simulink model "controlGPI_pos_3dof_conMI"  (R2023b)
settings: Solver=VariableStepAuto  StartTime=0.0  StopTime=tsim  FixedStep=1e-5  MaxStep=tstep  RelTol=1e-3
undefined symbols (not defined in the file): contr_robot_params, ddq, dq, MI_Contr1, MI_Contr2, MI_Contr3, MI_motor1, MI_motor2, MI_motor3, ndof, NN_Bspline_params, NN_RBF_params, nn_select, ns, Pc, q, q0, q_cero, q_eq, robot_params, sigbuilder_block, t_qeq_init, t_tr_init, t_trtr, tau_L, tau_L_mags, tr_muestra, Wc, Zc
libraries: mcbcontrolslib x6, spsRMSLib x6, simulink x2
(part 1 of 3)
settings Model: Creator=HP  LastModifiedBy=HP

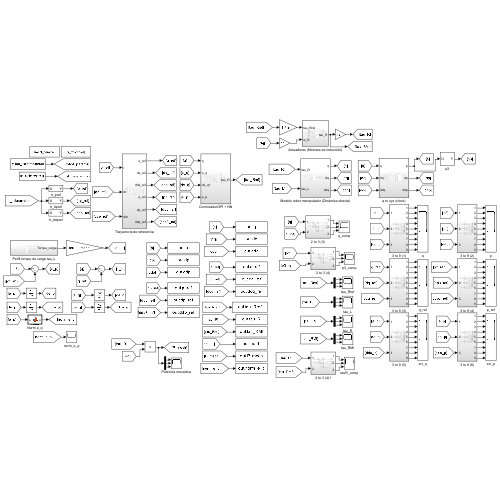
[thumbnail: Simulink's stored preview of the top-level diagram]
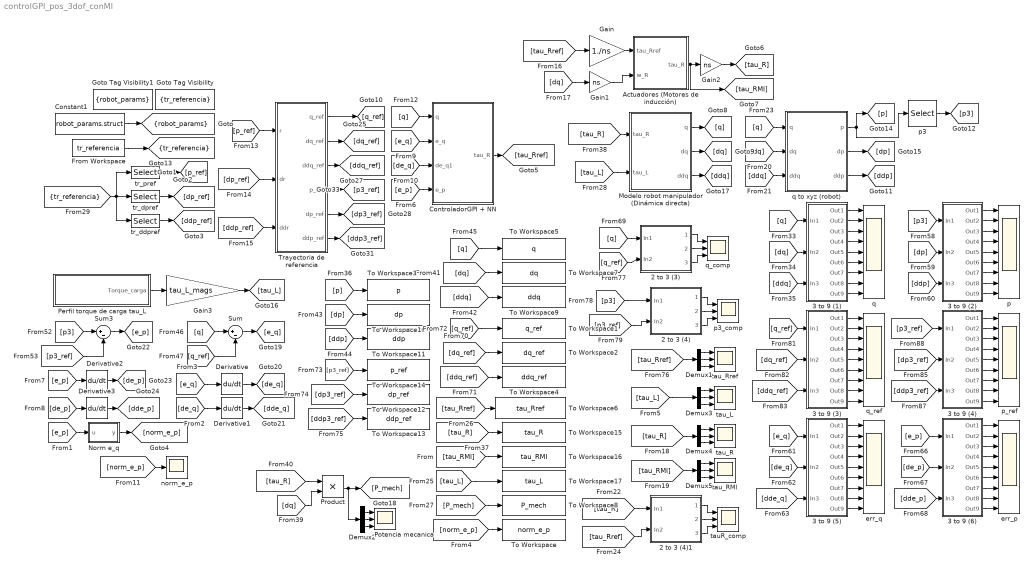
== system controlGPI_pos_3dof_conMI ==
  2 to 3 (3) : Subsystem
  2 to 3 (4) : Subsystem
  2 to 3 (4)1 : Subsystem
  3 to 9 (1) : Subsystem
  3 to 9 (2) : Subsystem
  3 to 9 (3) : Subsystem
  3 to 9 (4) : Subsystem
  3 to 9 (5) : Subsystem
  3 to 9 (6) : Subsystem
  Actuadores (Motores de inducción) : Subsystem
  Constant1 : Constant  Value=robot_params.struct  OutDataTypeStr=Bus: robot_params_bus
  ControladorGPI + NN : Subsystem
  Demux{1..5} (5 alike) : Demux  Outputs=3
  Derivative{,1..3} (4 alike) : Derivative
  From Workspace : FromWorkspace  VariableName=tr_referencia
  Gain : Gain  Gain=1./ns
  Gain1 : Gain  Gain=ns
  Gain2 : Gain  Gain=ns
  Gain3 : Gain  Gain=tau_L_mags
  Goto Tag Visibility : GotoTagVisibility  GotoTag=tr_referencia
  Goto Tag Visibility1 : GotoTagVisibility  GotoTag=robot_params
  Modelo robot manipulador (Dinámica directa) : Subsystem
  Norm e_q : MATLAB Function  TreatAsAtomicUnit=on
  Perfil torque de carga tau_L : Subsystem
  Potencia mecanica : Scope  NumInputPorts=3
  Product : Product
  Sum : Sum  Inputs=|+-
  Sum3 : Sum  Inputs=|+-
  To Workspace : ToWorkspace  VariableName=norm_e_p  SaveFormat=Timeseries  SampleTime=-1
  To Workspace1 : ToWorkspace  VariableName=q_ref  SaveFormat=Timeseries  SampleTime=-1
  To Workspace10 : ToWorkspace  VariableName=dp  SaveFormat=Timeseries  SampleTime=-1
  To Workspace11 : ToWorkspace  VariableName=ddp  SaveFormat=Timeseries  SampleTime=-1
  To Workspace12 : ToWorkspace  VariableName=dp_ref  SaveFormat=Timeseries  SampleTime=-1
  To Workspace13 : ToWorkspace  VariableName=ddp_ref  SaveFormat=Timeseries  SampleTime=-1
  To Workspace14 : ToWorkspace  VariableName=p_ref  SaveFormat=Timeseries  SampleTime=-1
  To Workspace15 : ToWorkspace  VariableName=tau_R  SaveFormat=Timeseries  SampleTime=-1
  To Workspace16 : ToWorkspace  VariableName=tau_RMI  SaveFormat=Timeseries  SampleTime=-1
  To Workspace17 : ToWorkspace  VariableName=tau_L  SaveFormat=Timeseries  SampleTime=-1
  To Workspace2 : ToWorkspace  VariableName=dq_ref  SaveFormat=Timeseries  SampleTime=-1
  To Workspace3 : ToWorkspace  VariableName=p  SaveFormat=Timeseries  SampleTime=-1
  To Workspace4 : ToWorkspace  VariableName=ddq_ref  SaveFormat=Timeseries  SampleTime=-1
  To Workspace5 : ToWorkspace  VariableName=q  SaveFormat=Timeseries  SampleTime=-1
  To Workspace6 : ToWorkspace  VariableName=tau_Rref  SaveFormat=Timeseries  SampleTime=-1
  To Workspace7 : ToWorkspace  VariableName=dq  SaveFormat=Timeseries  SampleTime=-1
  To Workspace8 : ToWorkspace  VariableName=P_mech  SaveFormat=Timeseries  SampleTime=-1
  To Workspace9 : ToWorkspace  VariableName=ddq  SaveFormat=Timeseries  SampleTime=-1
  Trayectoria de referencia : Subsystem
  err_p : Scope  NumInputPorts=9
  err_q : Scope  NumInputPorts=9
  norm_e_p : Scope
  p : Scope  NumInputPorts=9
  p3 : Selector  NumberOfDimensions=2  InputPortWidth=3  IndexOptions=Index vector (dialog),Index vector (dialog)  Indices=[1:3],3  OutputSizes=1,1
  p3_comp : Scope  NumInputPorts=3
  p_ref : Scope  NumInputPorts=9
  q : Scope  NumInputPorts=9
  q to xyz (robot) : Subsystem
  q_comp : Scope  NumInputPorts=3
  q_ref : Scope  NumInputPorts=9
  tauR_comp : Scope  NumInputPorts=3
  tau_L : Scope  NumInputPorts=3
  tau_R : Scope  NumInputPorts=3
  tau_RMI : Scope  NumInputPorts=3
  tau_Rref : Scope  NumInputPorts=3
  tr_ddpref : Selector  NumberOfDimensions=2  InputPortWidth=3  IndexOptions=Index vector (dialog),Index vector (dialog)  Indices=[7:9],1  OutputSizes=1,1
  tr_dpref : Selector  NumberOfDimensions=2  InputPortWidth=3  IndexOptions=Index vector (dialog),Index vector (dialog)  Indices=[4:6],1  OutputSizes=1,1
  tr_pref : Selector  NumberOfDimensions=2  InputPortWidth=3  IndexOptions=Index vector (dialog),Index vector (dialog)  Indices=[1:3],1  OutputSizes=1,1
  tag scope: robot_params=scoped, tr_referencia=scoped
  wires:
  From Workspace/1 -> [tr_referencia]
  Constant1/1 -> [robot_params]
  [tau_L] -> Modelo robot manipulador (Dinámica directa)/2(tau_L)
  [tau_R] -> Modelo robot manipulador (Dinámica directa)/1(tau_R)
  Modelo robot manipulador (Dinámica directa)/1(q) -> [q]
  Modelo robot manipulador (Dinámica directa)/2(dq) -> [dq]
  Modelo robot manipulador (Dinámica directa)/3(ddq) -> [ddq]
  [tr_referencia] -> tr_ddpref/1, tr_pref/1, tr_dpref/1
  tr_pref/1 -> [p_ref]
  tr_dpref/1 -> [dp_ref]
  tr_ddpref/1 -> [ddp_ref]
  3 to 9 (6)/4(Out4) -> err_p/4
  [e_q] -> 3 to 9 (5)/1(In1)
  3 to 9 (5)/6(Out6) -> err_q/6
  3 to 9 (5)/3(Out3) -> err_q/3
  3 to 9 (3)/6(Out6) -> q_ref/6
  3 to 9 (4)/4(Out4) -> p_ref/4
  Demux1/3 -> tau_Rref/3
  3 to 9 (5)/8(Out8) -> err_q/8
  [dq_ref] -> 3 to 9 (3)/2(In2)
  [dq] -> 3 to 9 (1)/2(In2)
  2 to 3 (4)/1(1) -> p3_comp/1
  3 to 9 (2)/6(Out6) -> p/6
  [tau_R] -> Product/1
  Product/1 -> Demux2/1, [P_mech]
  [q] -> 3 to 9 (1)/1(In1)
  3 to 9 (2)/3(Out3) -> p/3
  3 to 9 (1)/9(Out9) -> q/9
  [p3] -> 2 to 3 (4)/1(In1)
  2 to 3 (3)/2(2) -> q_comp/2
  [ddq_ref] -> 3 to 9 (3)/3(In3)
  3 to 9 (1)/5(Out5) -> q/5
  3 to 9 (3)/7(Out7) -> q_ref/7
  3 to 9 (2)/1(Out1) -> p/1
  3 to 9 (6)/1(Out1) -> err_p/1
  Demux2/1 -> Potencia mecanica/1
  3 to 9 (5)/9(Out9) -> err_q/9
  3 to 9 (3)/5(Out5) -> q_ref/5
  [dde_p] -> 3 to 9 (6)/3(In3)
  3 to 9 (5)/2(Out2) -> err_q/2
  3 to 9 (6)/8(Out8) -> err_p/8
  [p3] -> 3 to 9 (2)/1(In1)
  2 to 3 (3)/3(3) -> q_comp/3
  [tau_L] -> Demux3/1
  Demux2/2 -> Potencia mecanica/2
  3 to 9 (2)/2(Out2) -> p/2
  Demux1/2 -> tau_Rref/2
  3 to 9 (1)/6(Out6) -> q/6
  [de_q] -> 3 to 9 (5)/2(In2)
  3 to 9 (4)/6(Out6) -> p_ref/6
  [e_p] -> 3 to 9 (6)/1(In1)
  2 to 3 (4)/2(2) -> p3_comp/2
  3 to 9 (4)/7(Out7) -> p_ref/7
  3 to 9 (6)/5(Out5) -> err_p/5
  3 to 9 (4)/2(Out2) -> p_ref/2
  [dq] -> Product/2
  3 to 9 (1)/1(Out1) -> q/1
  3 to 9 (3)/8(Out8) -> q_ref/8
  3 to 9 (2)/9(Out9) -> p/9
  3 to 9 (3)/1(Out1) -> q_ref/1
  [de_p] -> 3 to 9 (6)/2(In2)
  [q] -> 2 to 3 (3)/1(In1)
  3 to 9 (1)/7(Out7) -> q/7
  3 to 9 (1)/2(Out2) -> q/2
  [q_ref] -> 2 to 3 (3)/2(In2)
  [tau_Rref] -> Demux1/1
  [ddq] -> 3 to 9 (1)/3(In3)
  3 to 9 (6)/2(Out2) -> err_p/2
  3 to 9 (4)/9(Out9) -> p_ref/9
  3 to 9 (5)/1(Out1) -> err_q/1
  3 to 9 (2)/4(Out4) -> p/4
  3 to 9 (2)/7(Out7) -> p/7
  3 to 9 (3)/4(Out4) -> q_ref/4
  3 to 9 (5)/7(Out7) -> err_q/7
  3 to 9 (4)/1(Out1) -> p_ref/1
  [p3_ref] -> 2 to 3 (4)/2(In2)
  [dde_q] -> 3 to 9 (5)/3(In3)
  3 to 9 (4)/8(Out8) -> p_ref/8
  3 to 9 (6)/6(Out6) -> err_p/6
  3 to 9 (1)/4(Out4) -> q/4
  3 to 9 (3)/3(Out3) -> q_ref/3
  3 to 9 (3)/9(Out9) -> q_ref/9
  2 to 3 (3)/1(1) -> q_comp/1
  3 to 9 (4)/5(Out5) -> p_ref/5
  [q_ref] -> 3 to 9 (3)/1(In1)
  2 to 3 (4)/3(3) -> p3_comp/3
  [dp3_ref] -> 3 to 9 (4)/2(In2)
  3 to 9 (1)/8(Out8) -> q/8
  [ddp3_ref] -> 3 to 9 (4)/3(In3)
  3 to 9 (5)/4(Out4) -> err_q/4
  3 to 9 (3)/2(Out2) -> q_ref/2
  3 to 9 (2)/5(Out5) -> p/5
  3 to 9 (5)/5(Out5) -> err_q/5
  3 to 9 (4)/3(Out3) -> p_ref/3
  Demux2/3 -> Potencia mecanica/3
  [p3_ref] -> 3 to 9 (4)/1(In1)
  3 to 9 (6)/3(Out3) -> err_p/3
  3 to 9 (2)/8(Out8) -> p/8
  3 to 9 (6)/9(Out9) -> err_p/9
  [ddp] -> 3 to 9 (2)/3(In3)
  [dp] -> 3 to 9 (2)/2(In2)
  Demux1/1 -> tau_Rref/1
  3 to 9 (1)/3(Out3) -> q/3
  3 to 9 (6)/7(Out7) -> err_p/7
  q to xyz (robot)/1(p) -> p3/1, [p]
  [dq] -> q to xyz (robot)/2(dq)
  [ddq] -> q to xyz (robot)/3(ddq)
  [q] -> To Workspace5/1
  [dq_ref] -> To Workspace2/1
  [q] -> q to xyz (robot)/1(q)
  [ddq] -> To Workspace9/1
  [p3_ref] -> To Workspace14/1
  [ddq_ref] -> To Workspace4/1
  [q_ref] -> To Workspace1/1
  q to xyz (robot)/2(dp) -> [dp]
  [dp] -> To Workspace10/1
  [dp3_ref] -> To Workspace12/1
  q to xyz (robot)/3(ddp) -> [ddp]
  [ddp] -> To Workspace11/1
  [p] -> To Workspace3/1
  [dq] -> To Workspace7/1
  p3/1 -> [p3]
  [ddp3_ref] -> To Workspace13/1
  [norm_e_p] -> norm_e_p/1
  Derivative2/1 -> [de_p]
  [e_p] -> Derivative2/1
  Derivative3/1 -> [dde_p]
  Derivative1/1 -> [dde_q]
  [e_q] -> Derivative/1
  [de_p] -> Derivative3/1
  Norm e_q/1(y) -> [norm_e_p]
  [e_p] -> Norm e_q/1(u)
  [p3_ref] -> Sum3/2
  Sum/1 -> [e_q]
  [de_q] -> Derivative1/1
  [q_ref] -> Sum/2
  [q] -> Sum/1
  Derivative/1 -> [de_q]
  [p3] -> Sum3/1
  Sum3/1 -> [e_p]
  [e_q] -> ControladorGPI + NN/2(e_q)
  [e_p] -> ControladorGPI + NN/4(e_p)
  [q] -> ControladorGPI + NN/1(q)
  [de_q] -> ControladorGPI + NN/3(de_q1)
  ControladorGPI + NN/1(tau_R) -> [tau_Rref]
  Demux3/3 -> tau_L/3
  Demux3/2 -> tau_L/2
  Demux3/1 -> tau_L/1
  [p_ref] -> Trayectoria de referencia/1(r)
  Trayectoria de referencia/6(ddp_ref) -> [ddp3_ref]
  Trayectoria de referencia/2(dq_ref) -> [dq_ref]
  [dp_ref] -> Trayectoria de referencia/2(dr)
  Trayectoria de referencia/5(dp_ref) -> [dp3_ref]
  Trayectoria de referencia/1(q_ref) -> [q_ref]
  Trayectoria de referencia/4(p_ref) -> [p3_ref]
  Trayectoria de referencia/3(ddq_ref) -> [ddq_ref]
  [ddp_ref] -> Trayectoria de referencia/3(ddr)
  Gain/1 -> Actuadores (Motores de inducción)/1(tau_Rref)
  Actuadores (Motores de inducción)/1(tau_R) -> [tau_RMI], Gain2/1
  Gain1/1 -> Actuadores (Motores de inducción)/2(w_R)
  Gain2/1 -> [tau_R]
  [tau_Rref] -> Gain/1
  [dq] -> Gain1/1
  Demux4/3 -> tau_R/3
  Demux4/1 -> tau_R/1
  Demux4/2 -> tau_R/2
  [tau_R] -> Demux4/1
  [tau_RMI] -> Demux5/1
  Demux5/2 -> tau_RMI/2
  Demux5/3 -> tau_RMI/3
  Demux5/1 -> tau_RMI/1
  2 to 3 (4)1/3(3) -> tauR_comp/3
  2 to 3 (4)1/2(2) -> tauR_comp/2
  2 to 3 (4)1/1(1) -> tauR_comp/1
  [tau_R] -> 2 to 3 (4)1/1(In1)
  [tau_Rref] -> 2 to 3 (4)1/2(In2)
  Perfil torque de carga tau_L/1(Torque_carga) -> Gain3/1
  Gain3/1 -> [tau_L]
  [P_mech] -> To Workspace8/1
  [tau_Rref] -> To Workspace6/1
  [tau_RMI] -> To Workspace16/1
  [tau_R] -> To Workspace15/1
  [tau_L] -> To Workspace17/1
  [norm_e_p] -> To Workspace/1

== system controlGPI_pos_3dof_conMI/2 to 3 (3) ==
  In1 : Inport
  In2 : Inport  Port=2
  Demux3 : Demux  Outputs=3
  Demux4 : Demux  Outputs=3
  Mux10 : Mux  Inputs=2
  Mux8 : Mux  Inputs=2
  Mux9 : Mux  Inputs=2
  1 : Outport
  2 : Outport  Port=2
  3 : Outport  Port=3
  wires:
  Demux4/3 -> Mux10/2
  Demux3/1 -> Mux8/1
  Demux3/2 -> Mux9/1
  Mux9/1 -> 2/1
  Demux4/2 -> Mux9/2
  Demux4/1 -> Mux8/2
  Demux3/3 -> Mux10/1
  Mux8/1 -> 1/1
  Mux10/1 -> 3/1
  In1/1 -> Demux3/1
  In2/1 -> Demux4/1

== system controlGPI_pos_3dof_conMI/2 to 3 (4) ==
  In1 : Inport
  In2 : Inport  Port=2
  Demux3 : Demux  Outputs=3
  Demux4 : Demux  Outputs=3
  Mux10 : Mux  Inputs=2
  Mux8 : Mux  Inputs=2
  Mux9 : Mux  Inputs=2
  1 : Outport
  2 : Outport  Port=2
  3 : Outport  Port=3
  wires:
  Demux4/3 -> Mux10/2
  Demux3/1 -> Mux8/1
  Demux3/2 -> Mux9/1
  Mux9/1 -> 2/1
  Demux4/2 -> Mux9/2
  Demux4/1 -> Mux8/2
  Demux3/3 -> Mux10/1
  Mux8/1 -> 1/1
  Mux10/1 -> 3/1
  In1/1 -> Demux3/1
  In2/1 -> Demux4/1

== system controlGPI_pos_3dof_conMI/2 to 3 (4)1 ==
  In1 : Inport
  In2 : Inport  Port=2
  Demux3 : Demux  Outputs=3
  Demux4 : Demux  Outputs=3
  Mux10 : Mux  Inputs=2
  Mux8 : Mux  Inputs=2
  Mux9 : Mux  Inputs=2
  1 : Outport
  2 : Outport  Port=2
  3 : Outport  Port=3
  wires:
  Demux4/3 -> Mux10/2
  Demux3/1 -> Mux8/1
  Demux3/2 -> Mux9/1
  Mux9/1 -> 2/1
  Demux4/2 -> Mux9/2
  Demux4/1 -> Mux8/2
  Demux3/3 -> Mux10/1
  Mux8/1 -> 1/1
  Mux10/1 -> 3/1
  In1/1 -> Demux3/1
  In2/1 -> Demux4/1

== system controlGPI_pos_3dof_conMI/3 to 9 (1) ==
  In1 : Inport
  In2 : Inport  Port=2
  In3 : Inport  Port=3
  Demux2 : Demux  Outputs=3
  Demux3 : Demux  Outputs=3
  Demux4 : Demux  Outputs=3
  Out1 : Outport
  Out2 : Outport  Port=2
  Out3 : Outport  Port=3
  Out4 : Outport  Port=4
  Out5 : Outport  Port=5
  Out6 : Outport  Port=6
  Out7 : Outport  Port=7
  Out8 : Outport  Port=8
  Out9 : Outport  Port=9
  wires:
  In3/1 -> Demux4/1
  Demux4/1 -> Out3/1
  Demux2/1 -> Out1/1
  Demux3/3 -> Out8/1
  Demux3/2 -> Out5/1
  Demux3/1 -> Out2/1
  In1/1 -> Demux2/1
  Demux2/3 -> Out7/1
  Demux4/3 -> Out9/1
  Demux4/2 -> Out6/1
  Demux2/2 -> Out4/1
  In2/1 -> Demux3/1

== system controlGPI_pos_3dof_conMI/3 to 9 (2) ==
  In1 : Inport
  In2 : Inport  Port=2
  In3 : Inport  Port=3
  Demux2 : Demux  Outputs=3
  Demux3 : Demux  Outputs=3
  Demux4 : Demux  Outputs=3
  Out1 : Outport
  Out2 : Outport  Port=2
  Out3 : Outport  Port=3
  Out4 : Outport  Port=4
  Out5 : Outport  Port=5
  Out6 : Outport  Port=6
  Out7 : Outport  Port=7
  Out8 : Outport  Port=8
  Out9 : Outport  Port=9
  wires:
  In3/1 -> Demux4/1
  Demux4/1 -> Out3/1
  Demux2/1 -> Out1/1
  Demux3/3 -> Out8/1
  Demux3/2 -> Out5/1
  Demux3/1 -> Out2/1
  In1/1 -> Demux2/1
  Demux2/3 -> Out7/1
  Demux4/3 -> Out9/1
  Demux4/2 -> Out6/1
  Demux2/2 -> Out4/1
  In2/1 -> Demux3/1

== system controlGPI_pos_3dof_conMI/3 to 9 (3) ==
  In1 : Inport
  In2 : Inport  Port=2
  In3 : Inport  Port=3
  Demux2 : Demux  Outputs=3
  Demux3 : Demux  Outputs=3
  Demux4 : Demux  Outputs=3
  Out1 : Outport
  Out2 : Outport  Port=2
  Out3 : Outport  Port=3
  Out4 : Outport  Port=4
  Out5 : Outport  Port=5
  Out6 : Outport  Port=6
  Out7 : Outport  Port=7
  Out8 : Outport  Port=8
  Out9 : Outport  Port=9
  wires:
  In3/1 -> Demux4/1
  Demux4/1 -> Out3/1
  Demux2/1 -> Out1/1
  Demux3/3 -> Out8/1
  Demux3/2 -> Out5/1
  Demux3/1 -> Out2/1
  In1/1 -> Demux2/1
  Demux2/3 -> Out7/1
  Demux4/3 -> Out9/1
  Demux4/2 -> Out6/1
  Demux2/2 -> Out4/1
  In2/1 -> Demux3/1

== system controlGPI_pos_3dof_conMI/3 to 9 (4) ==
  In1 : Inport
  In2 : Inport  Port=2
  In3 : Inport  Port=3
  Demux2 : Demux  Outputs=3
  Demux3 : Demux  Outputs=3
  Demux4 : Demux  Outputs=3
  Out1 : Outport
  Out2 : Outport  Port=2
  Out3 : Outport  Port=3
  Out4 : Outport  Port=4
  Out5 : Outport  Port=5
  Out6 : Outport  Port=6
  Out7 : Outport  Port=7
  Out8 : Outport  Port=8
  Out9 : Outport  Port=9
  wires:
  In3/1 -> Demux4/1
  Demux4/1 -> Out3/1
  Demux2/1 -> Out1/1
  Demux3/3 -> Out8/1
  Demux3/2 -> Out5/1
  Demux3/1 -> Out2/1
  In1/1 -> Demux2/1
  Demux2/3 -> Out7/1
  Demux4/3 -> Out9/1
  Demux4/2 -> Out6/1
  Demux2/2 -> Out4/1
  In2/1 -> Demux3/1

== system controlGPI_pos_3dof_conMI/3 to 9 (5) ==
  In1 : Inport
  In2 : Inport  Port=2
  In3 : Inport  Port=3
  Demux2 : Demux  Outputs=3
  Demux3 : Demux  Outputs=3
  Demux4 : Demux  Outputs=3
  Out1 : Outport
  Out2 : Outport  Port=2
  Out3 : Outport  Port=3
  Out4 : Outport  Port=4
  Out5 : Outport  Port=5
  Out6 : Outport  Port=6
  Out7 : Outport  Port=7
  Out8 : Outport  Port=8
  Out9 : Outport  Port=9
  wires:
  In3/1 -> Demux4/1
  Demux4/1 -> Out3/1
  Demux2/1 -> Out1/1
  Demux3/3 -> Out8/1
  Demux3/2 -> Out5/1
  Demux3/1 -> Out2/1
  In1/1 -> Demux2/1
  Demux2/3 -> Out7/1
  Demux4/3 -> Out9/1
  Demux4/2 -> Out6/1
  Demux2/2 -> Out4/1
  In2/1 -> Demux3/1

== system controlGPI_pos_3dof_conMI/3 to 9 (6) ==
  In1 : Inport
  In2 : Inport  Port=2
  In3 : Inport  Port=3
  Demux2 : Demux  Outputs=3
  Demux3 : Demux  Outputs=3
  Demux4 : Demux  Outputs=3
  Out1 : Outport
  Out2 : Outport  Port=2
  Out3 : Outport  Port=3
  Out4 : Outport  Port=4
  Out5 : Outport  Port=5
  Out6 : Outport  Port=6
  Out7 : Outport  Port=7
  Out8 : Outport  Port=8
  Out9 : Outport  Port=9
  wires:
  In3/1 -> Demux4/1
  Demux4/1 -> Out3/1
  Demux2/1 -> Out1/1
  Demux3/3 -> Out8/1
  Demux3/2 -> Out5/1
  Demux3/1 -> Out2/1
  In1/1 -> Demux2/1
  Demux2/3 -> Out7/1
  Demux4/3 -> Out9/1
  Demux4/2 -> Out6/1
  Demux2/2 -> Out4/1
  In2/1 -> Demux3/1

== system controlGPI_pos_3dof_conMI/Actuadores (Motores de inducción) ==
  tau_Rref : Inport
  w_R : Inport  Port=2
  Demux : Demux  Outputs=3
  Demux3 : Demux  Outputs=3
  MI1 + PBC Torque Controller : Subsystem
  MI2 + PBC Torque Controller : Subsystem
  MI3 + PBC Torque Controller : Subsystem
  Mux : Mux  Inputs=3
  tau_R : Outport
  wires:
  Demux3/1 -> MI1 + PBC Torque Controller/2(dq)
  Demux/1 -> MI1 + PBC Torque Controller/1(tau_Rref)
  MI1 + PBC Torque Controller/1(tau_R) -> Mux/1
  Demux3/3 -> MI3 + PBC Torque Controller/2(dq)
  MI2 + PBC Torque Controller/1(tau_R) -> Mux/2
  MI3 + PBC Torque Controller/1(tau_R) -> Mux/3
  Demux3/2 -> MI2 + PBC Torque Controller/2(dq)
  Demux/3 -> MI3 + PBC Torque Controller/1(tau_Rref)
  Demux/2 -> MI2 + PBC Torque Controller/1(tau_Rref)
  tau_Rref/1 -> Demux/1
  w_R/1 -> Demux3/1
  Mux/1 -> tau_R/1

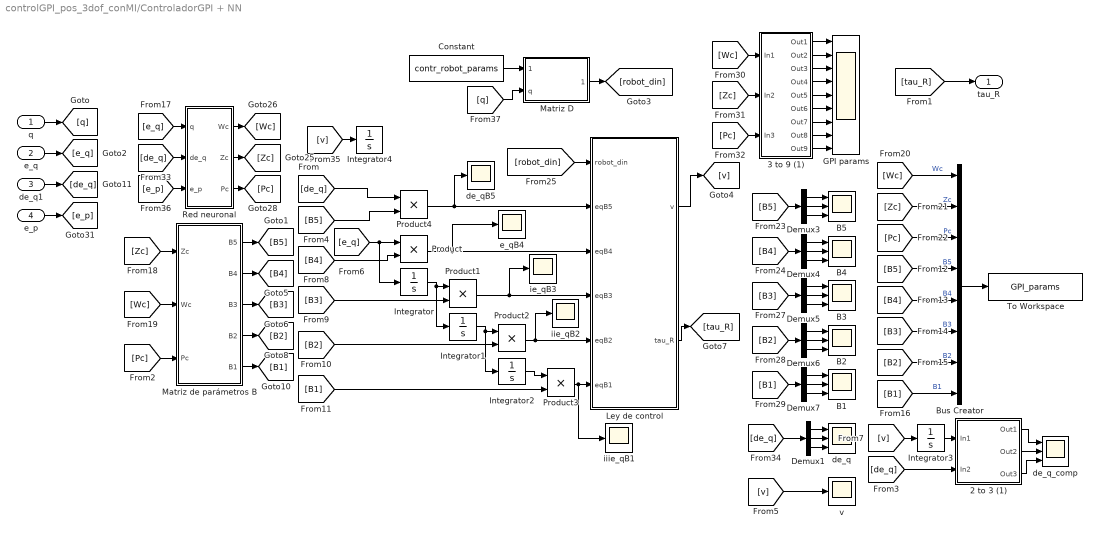
== system controlGPI_pos_3dof_conMI/ControladorGPI + NN ==
  q : Inport
  e_q : Inport  Port=2
  de_q1 : Inport  Port=3
  e_p : Inport  Port=4
  2 to 3 (1) : Subsystem
  3 to 9 (1) : Subsystem
  B{1..5} (5 alike) : Scope  NumInputPorts=3
  Bus Creator : BusCreator  Inputs=8
  Constant : Constant  Value=contr_robot_params  OutDataTypeStr=Bus: robot_params_bus
  Demux{1,3..7} (6 alike) : Demux  Outputs=3
  GPI params : Scope  NumInputPorts=9
  Integrator{,1..4} (5 alike) : Integrator
  Ley de control : MATLAB Function  TreatAsAtomicUnit=on
  Matriz D : MATLAB Function  TreatAsAtomicUnit=on
  Matriz de parámetros B : MATLAB Function  TreatAsAtomicUnit=on
  Product{,1..4} (5 alike) : Product
  Red neuronal : Subsystem
  To Workspace : ToWorkspace  VariableName=GPI_params  SaveFormat=Timeseries  SampleTime=-1
  de_q : Scope  NumInputPorts=3
  de_qB5 : Scope
  de_q_comp : Scope  NumInputPorts=3
  e_qB4 : Scope
  ie_qB3 : Scope
  iie_qB2 : Scope
  iiie_qB1 : Scope
  v : Scope
  tau_R : Outport
  wires:
  Ley de control/2(tau_R) -> [tau_R]
  [tau_R] -> tau_R/1
  e_q/1 -> [e_q]
  [e_q] -> Integrator/1, Product/1
  Integrator/1 -> Integrator1/1, Product1/1
  Integrator1/1 -> Integrator2/1, Product2/1
  Integrator2/1 -> Product3/1
  Product3/1 -> iiie_qB1/1, Ley de control/6(eqB1)
  Product2/1 -> iie_qB2/1, Ley de control/5(eqB2)
  Product1/1 -> ie_qB3/1, Ley de control/4(eqB3)
  Product/1 -> e_qB4/1, Ley de control/3(eqB4)
  Ley de control/1(v) -> [v]
  Product4/1 -> de_qB5/1, Ley de control/2(eqB5)
  [Zc] -> Matriz de parámetros B/1(Zc)
  [Wc] -> Matriz de parámetros B/2(Wc)
  [Pc] -> Matriz de parámetros B/3(Pc)
  Matriz de parámetros B/1(B5) -> [B5]
  Matriz de parámetros B/2(B4) -> [B4]
  Matriz de parámetros B/3(B3) -> [B3]
  Matriz de parámetros B/4(B2) -> [B2]
  Matriz de parámetros B/5(B1) -> [B1]
  [B5] -> Product4/2
  [B4] -> Product/2
  [B3] -> Product1/2
  [B2] -> Product2/2
  [B1] -> Product3/2
  Bus Creator/1 -> To Workspace/1
  [Wc] -> Bus Creator/1  "Wc"
  [Zc] -> Bus Creator/2  "Zc"
  [Pc] -> Bus Creator/3  "Pc"
  [B5] -> Bus Creator/4  "B5"
  [B4] -> Bus Creator/5  "B4"
  [B3] -> Bus Creator/6  "B3"
  [B2] -> Bus Creator/7  "B2"
  [B1] -> Bus Creator/8  "B1"
  Demux3/2 -> B5/2
  Demux3/1 -> B5/1
  [B5] -> Demux3/1
  Demux4/2 -> B4/2
  Demux4/1 -> B4/1
  [B4] -> Demux4/1
  Demux5/1 -> B3/1
  Demux5/2 -> B3/2
  [B3] -> Demux5/1
  Demux6/1 -> B2/1
  Demux6/2 -> B2/2
  [B2] -> Demux6/1
  Demux7/1 -> B1/1
  Demux7/2 -> B1/2
  [B1] -> Demux7/1
  Red neuronal/2(Zc) -> [Zc]
  Red neuronal/1(Wc) -> [Wc]
  Red neuronal/3(Pc) -> [Pc]
  [de_q] -> Red neuronal/2(de_q)
  [e_q] -> Red neuronal/1(q)
  [de_q] -> Demux1/1
  Demux1/1 -> de_q/1
  Demux1/2 -> de_q/2
  de_q1/1 -> [de_q]
  e_p/1 -> [e_p]
  [e_p] -> Red neuronal/3(e_p)
  [robot_din] -> Ley de control/1(robot_din)
  q/1 -> [q]
  [v] -> Integrator3/1
  Integrator3/1 -> 2 to 3 (1)/1(In1)
  [de_q] -> 2 to 3 (1)/2(In2)
  [v] -> v/1
  [v] -> Integrator4/1
  [de_q] -> Product4/1
  3 to 9 (1)/6(Out6) -> GPI params/6
  3 to 9 (1)/9(Out9) -> GPI params/9
  3 to 9 (1)/2(Out2) -> GPI params/2
  3 to 9 (1)/8(Out8) -> GPI params/8
  [Pc] -> 3 to 9 (1)/3(In3)
  3 to 9 (1)/1(Out1) -> GPI params/1
  [Wc] -> 3 to 9 (1)/1(In1)
  3 to 9 (1)/7(Out7) -> GPI params/7
  3 to 9 (1)/4(Out4) -> GPI params/4
  3 to 9 (1)/3(Out3) -> GPI params/3
  [Zc] -> 3 to 9 (1)/2(In2)
  3 to 9 (1)/5(Out5) -> GPI params/5
  2 to 3 (1)/1(Out1) -> de_q_comp/1
  2 to 3 (1)/2(Out2) -> de_q_comp/2
  2 to 3 (1)/3(Out3) -> de_q_comp/3
  Demux3/3 -> B5/3
  Demux4/3 -> B4/3
  Demux5/3 -> B3/3
  Demux6/3 -> B2/3
  Demux7/3 -> B1/3
  Demux1/3 -> de_q/3
  Constant/1 -> Matriz D/1(robot_params)
  [q] -> Matriz D/2(q)
  Matriz D/1(robot_din) -> [robot_din]

== system controlGPI_pos_3dof_conMI/Modelo robot manipulador (Dinámica directa) ==
  tau_R : Inport
  tau_L : Inport  Port=2
  Dinámica directa : MATLAB Function  TreatAsAtomicUnit=on
  int_ddq : Integrator  InitialCondition=q_cero
  int_dq : Integrator  InitialCondition=q_eq
  q : Outport
  dq : Outport  Port=2
  ddq : Outport  Port=3
  wires:
  [tau_L] -> Dinámica directa/5(tau_L)
  int_ddq/1 -> [dq], int_dq/1
  [robot_params] -> Dinámica directa/1(robot_params)
  [dq] -> Dinámica directa/3(dq)
  int_dq/1 -> [q]
  [tau_R] -> Dinámica directa/4(tau_R)
  Dinámica directa/1(ddq) -> int_ddq/1, [ddq]
  [q] -> q/1
  [dq] -> dq/1
  [ddq] -> ddq/1
  tau_R/1 -> [tau_R]
  tau_L/1 -> [tau_L]
  [q] -> Dinámica directa/2(q)

== system controlGPI_pos_3dof_conMI/Perfil torque de carga tau_L ==
  Bus Selector : BusSelector  OutputSignals=sel_perfil
  Bus Selector1 : BusSelector  OutputSignals=sel_perfil
  Constant17 : Constant  Value=tau_L.perfiles  OutDataTypeStr=Bus: Perfil_bus
  If : If  IfExpression=u1 == 1  ElseIfExpressions=u1 == 2,u1 == 3,u1 == 4,u1 == 5,u1 == 6,u1 == 7,u1 == 8
  If Action Subsystem : Subsystem  TreatAsAtomicUnit=on
  If Action Subsystem1 : Subsystem  TreatAsAtomicUnit=on
  If Action Subsystem2 : Subsystem  TreatAsAtomicUnit=on
  If Action Subsystem3 : Subsystem  TreatAsAtomicUnit=on
  If Action Subsystem4 : Subsystem  TreatAsAtomicUnit=on
  If Action Subsystem5 : Subsystem  TreatAsAtomicUnit=on
  If Action Subsystem6 : Subsystem  TreatAsAtomicUnit=on
  If Action Subsystem7 : Subsystem  TreatAsAtomicUnit=on
  tau_L : MultiPortSwitch  Inputs=9  SaturateOnIntegerOverflow=off  InputSameDT=off
  Torque_carga : Outport
  wires:
  tau_L/1 -> Torque_carga/1
  [ramp] -> tau_L/4
  [trEsca] -> tau_L/7
  [pol7] -> tau_L/6
  [sen] -> tau_L/5
  [esca] -> tau_L/3
  Constant17/1 -> [perfil_params]
  [ts] -> tau_L/8
  [tr15segs] -> tau_L/9
  Bus Selector/1 -> tau_L/1  "<sel_perfil>"
  [perfil_params] -> Bus Selector/1
  If Action Subsystem/1(sen) -> [sen]
  [perfil_params] -> Bus Selector1/1
  Bus Selector1/1 -> If/1  "<sel_perfil>"
  If/4 -> If Action Subsystem/Action
  If Action Subsystem1/1(cero) -> [cero]
  [cero] -> tau_L/2
  [perfil_params] -> If Action Subsystem/1(perfil_params)
  If/1 -> If Action Subsystem1/Action
  If Action Subsystem2/1(esca) -> [esca]
  If/2 -> If Action Subsystem2/Action
  If Action Subsystem3/1(ramp) -> [ramp]
  If/3 -> If Action Subsystem3/Action
  [perfil_params] -> If Action Subsystem4/1(perfil_params)
  If/5 -> If Action Subsystem4/Action
  If Action Subsystem4/1(pol7) -> [pol7]
  If Action Subsystem5/1(trEsca) -> [trEsca]
  [perfil_params] -> If Action Subsystem5/1(perfil_params)
  If Action Subsystem6/1(ts) -> [ts]
  If/6 -> If Action Subsystem5/Action
  If/7 -> If Action Subsystem6/Action
  If Action Subsystem7/1(tr15segs) -> [tr15segs]
  If/8 -> If Action Subsystem7/Action
  [perfil_params] -> If Action Subsystem7/1(perfil_params)

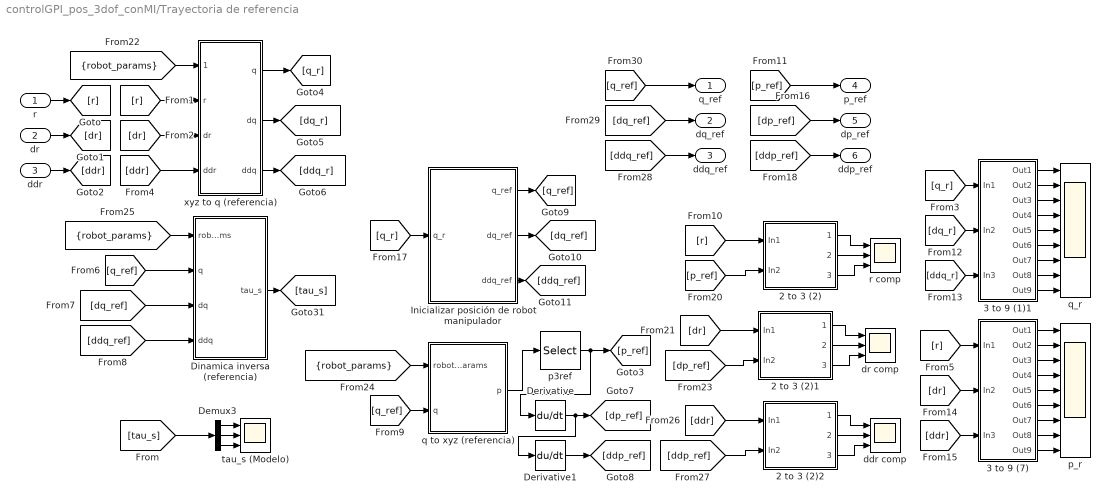
== system controlGPI_pos_3dof_conMI/Trayectoria de referencia ==
  r : Inport
  dr : Inport  Port=2
  ddr : Inport  Port=3
  2 to 3 (2) : Subsystem
  2 to 3 (2)1 : Subsystem
  2 to 3 (2)2 : Subsystem
  3 to 9 (1)1 : Subsystem
  3 to 9 (7) : Subsystem
  Demux3 : Demux  Outputs=3
  Derivative : Derivative
  Derivative1 : Derivative
  Dinamica inversa (referencia) : MATLAB Function  TreatAsAtomicUnit=on
  Inicializar posición de robot manipulador : Subsystem
  ddr comp : Scope  NumInputPorts=3
  dr comp : Scope  NumInputPorts=3
  p3ref : Selector  NumberOfDimensions=2  InputPortWidth=3  IndexOptions=Index vector (dialog),Index vector (dialog)  Indices=[1:3],3  OutputSizes=1,1
  p_r : Scope  NumInputPorts=9
  q to xyz (referencia) : MATLAB Function  TreatAsAtomicUnit=on
  q_r : Scope  NumInputPorts=9
  r comp : Scope  NumInputPorts=3
  tau_s (Modelo) : Scope  NumInputPorts=3
  xyz to q (referencia) : MATLAB Function  TreatAsAtomicUnit=on
  q_ref : Outport
  dq_ref : Outport  Port=2
  ddq_ref : Outport  Port=3
  p_ref : Outport  Port=4
  dp_ref : Outport  Port=5
  ddp_ref : Outport  Port=6
  wires:
  xyz to q (referencia)/1(q) -> [q_r]
  [robot_params] -> xyz to q (referencia)/1(robot_params)
  [dq_ref] -> Dinamica inversa (referencia)/3(dq)
  [q_ref] -> Dinamica inversa (referencia)/2(q)
  [q_ref] -> q to xyz (referencia)/2(q)
  [r] -> xyz to q (referencia)/2(r)
  xyz to q (referencia)/2(dq) -> [dq_r]
  q to xyz (referencia)/1(p) -> p3ref/1
  [robot_params] -> Dinamica inversa (referencia)/1(robot_params)
  Dinamica inversa (referencia)/1(tau_s) -> [tau_s]
  xyz to q (referencia)/3(ddq) -> [ddq_r]
  [ddq_ref] -> Dinamica inversa (referencia)/4(ddq)
  [ddr] -> xyz to q (referencia)/4(ddr)
  [dr] -> xyz to q (referencia)/3(dr)
  r/1 -> [r]
  dr/1 -> [dr]
  ddr/1 -> [ddr]
  Derivative/1 -> Derivative1/1, [dp_ref]
  [tau_s] -> Demux3/1
  [q_r] -> Inicializar posición de robot manipulador/1(q_r)
  [robot_params] -> q to xyz (referencia)/1(robot_params)
  2 to 3 (2)/2(2) -> r comp/2
  p3ref/1 -> [p_ref], Derivative/1
  2 to 3 (2)/1(1) -> r comp/1
  [r] -> 2 to 3 (2)/1(In1)
  2 to 3 (2)/3(3) -> r comp/3
  [p_ref] -> p_ref/1
  Derivative1/1 -> [ddp_ref]
  [dp_ref] -> dp_ref/1
  [ddp_ref] -> ddp_ref/1
  [p_ref] -> 2 to 3 (2)/2(In2)
  [dp_ref] -> 2 to 3 (2)1/2(In2)
  2 to 3 (2)1/2(2) -> dr comp/2
  2 to 3 (2)1/1(1) -> dr comp/1
  [dr] -> 2 to 3 (2)1/1(In1)
  2 to 3 (2)1/3(3) -> dr comp/3
  [ddp_ref] -> 2 to 3 (2)2/2(In2)
  2 to 3 (2)2/2(2) -> ddr comp/2
  2 to 3 (2)2/1(1) -> ddr comp/1
  [ddr] -> 2 to 3 (2)2/1(In1)
  2 to 3 (2)2/3(3) -> ddr comp/3
  Inicializar posición de robot manipulador/1(q_ref) -> [q_ref]
  Inicializar posición de robot manipulador/2(dq_ref) -> [dq_ref]
  Inicializar posición de robot manipulador/3(ddq_ref) -> [ddq_ref]
  [ddq_ref] -> ddq_ref/1
  [dq_ref] -> dq_ref/1
  [q_ref] -> q_ref/1
  3 to 9 (7)/4(Out4) -> p_r/4
  3 to 9 (7)/5(Out5) -> p_r/5
  3 to 9 (7)/8(Out8) -> p_r/8
  [ddr] -> 3 to 9 (7)/3(In3)
  [dq_r] -> 3 to 9 (1)1/2(In2)
  3 to 9 (7)/1(Out1) -> p_r/1
  3 to 9 (1)1/5(Out5) -> q_r/5
  3 to 9 (1)1/3(Out3) -> q_r/3
  3 to 9 (7)/3(Out3) -> p_r/3
  [r] -> 3 to 9 (7)/1(In1)
  3 to 9 (1)1/4(Out4) -> q_r/4
  3 to 9 (1)1/6(Out6) -> q_r/6
  [q_r] -> 3 to 9 (1)1/1(In1)
  3 to 9 (1)1/8(Out8) -> q_r/8
  3 to 9 (7)/7(Out7) -> p_r/7
  3 to 9 (1)1/7(Out7) -> q_r/7
  3 to 9 (1)1/1(Out1) -> q_r/1
  3 to 9 (1)1/2(Out2) -> q_r/2
  [dr] -> 3 to 9 (7)/2(In2)
  3 to 9 (7)/6(Out6) -> p_r/6
  3 to 9 (7)/2(Out2) -> p_r/2
  3 to 9 (7)/9(Out9) -> p_r/9
  3 to 9 (1)1/9(Out9) -> q_r/9
  [ddq_r] -> 3 to 9 (1)1/3(In3)
  Demux3/2 -> tau_s (Modelo)/2
  Demux3/1 -> tau_s (Modelo)/1
  Demux3/3 -> tau_s (Modelo)/3

== system controlGPI_pos_3dof_conMI/q to xyz (robot) ==
  q : Inport
  dq : Inport  Port=2
  ddq : Inport  Port=3
  Data Store Memory : DataStoreMemory  DataStoreName=q  WriteAfterWriteMsg=warning  InitialValue=zeros(size(q(:,1)))  ShowAdditionalParam=off
  Data Store Memory1 : DataStoreMemory  DataStoreName=dq  WriteAfterWriteMsg=warning  InitialValue=zeros(size(dq(:,1)))  ShowAdditionalParam=off
  Data Store Memory2 : DataStoreMemory  DataStoreName=ddq  WriteAfterWriteMsg=warning  InitialValue=zeros(size(ddq(:,1)))  ShowAdditionalParam=off
  Data Store Read : DataStoreRead  DataStoreName=q  IndexOptions=Index vector (dialog)  Indices=1  OutputSizes=1
  Data Store Read1 : DataStoreRead  DataStoreName=dq  IndexOptions=Index vector (dialog)  Indices=1  OutputSizes=1
  Data Store Read2 : DataStoreRead  DataStoreName=ddq  IndexOptions=Index vector (dialog)  Indices=1  OutputSizes=1
  Data Store Write : DataStoreWrite  DataStoreName=q  IndexOptions=Index vector (dialog)  Indices=1  OutputSizes=1
  Data Store Write1 : DataStoreWrite  DataStoreName=dq  IndexOptions=Index vector (dialog)  Indices=1  OutputSizes=1
  Data Store Write2 : DataStoreWrite  DataStoreName=ddq  IndexOptions=Index vector (dialog)  Indices=1  OutputSizes=1
  q to xyz (referencia) : MATLAB Function  TreatAsAtomicUnit=on
  p : Outport
  dp : Outport  Port=2
  ddp : Outport  Port=3
  wires:
  q/1 -> Data Store Write/1
  ddq/1 -> Data Store Write2/1
  dq/1 -> Data Store Write1/1
  Data Store Read/1 -> q to xyz (referencia)/2(q)
  Data Store Read1/1 -> q to xyz (referencia)/3(dq)
  Data Store Read2/1 -> q to xyz (referencia)/4(ddq)
  q to xyz (referencia)/1(p) -> p/1
  q to xyz (referencia)/2(dp) -> dp/1
  q to xyz (referencia)/3(ddp) -> ddp/1
  [robot_params] -> q to xyz (referencia)/1(robot_params)

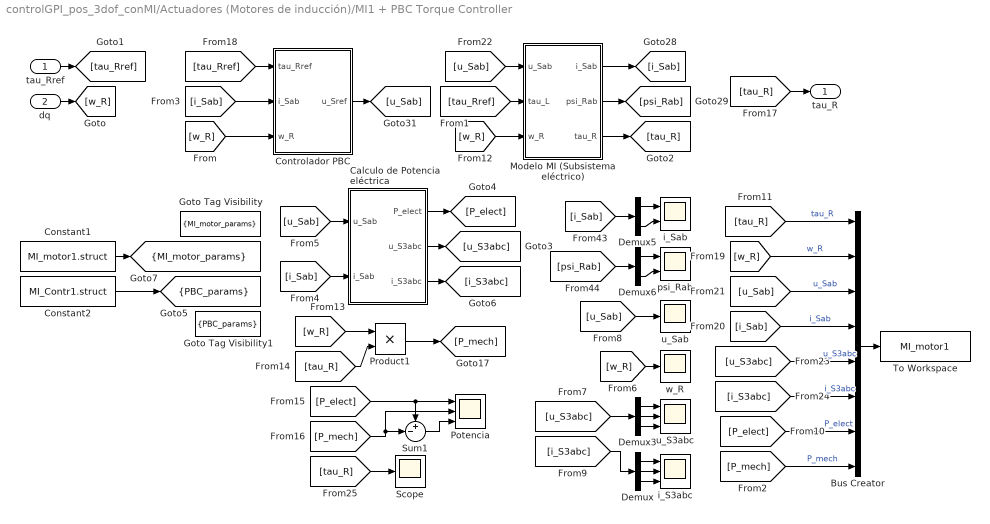
== system controlGPI_pos_3dof_conMI/Actuadores (Motores de inducción)/MI1 + PBC Torque Controller ==
  tau_Rref : Inport
  dq : Inport  Port=2
  Bus Creator : BusCreator  Inputs=8
  Calculo de Potencia eléctrica : Subsystem
  Constant1 : Constant  Value=MI_motor1.struct  OutDataTypeStr=Bus: MI_bus
  Constant2 : Constant  Value=MI_Contr1.struct  OutDataTypeStr=Bus: PBC_bus
  Controlador PBC : Subsystem
  Demux : Demux  Outputs=3
  Demux3 : Demux  Outputs=3
  Demux5 : Demux  Outputs=2
  Demux6 : Demux  Outputs=2
  Goto Tag Visibility : GotoTagVisibility  GotoTag=MI_motor_params
  Goto Tag Visibility1 : GotoTagVisibility  GotoTag=PBC_params
  Modelo MI (Subsistema eléctrico) : Subsystem
  Potencia : Scope  NumInputPorts=3
  Product1 : Product
  Scope : Scope
  Sum1 : Sum  Inputs=+-|
  To Workspace : ToWorkspace  VariableName=MI_motor1  SaveFormat=Timeseries  SampleTime=-1
  i_S3abc : Scope  NumInputPorts=3
  i_Sab : Scope  NumInputPorts=2
  psi_Rab : Scope  NumInputPorts=2
  u_S3abc : Scope  NumInputPorts=3
  u_Sab : Scope
  w_R : Scope
  tau_R : Outport
  tag scope: MI_motor_params=scoped, PBC_params=scoped
  wires:
  Modelo MI (Subsistema eléctrico)/2(psi_Rab) -> [psi_Rab]
  [u_Sab] -> Modelo MI (Subsistema eléctrico)/1(u_Sab)
  [i_Sab] -> Controlador PBC/2(i_Sab)
  Controlador PBC/1(u_Sref) -> [u_Sab]
  [w_R] -> Controlador PBC/3(w_R)
  [tau_Rref] -> Modelo MI (Subsistema eléctrico)/2(tau_L)
  Calculo de Potencia eléctrica/2(u_S3abc) -> [u_S3abc]
  Calculo de Potencia eléctrica/1(P_elect) -> [P_elect]
  Demux5/1 -> i_Sab/1
  [w_R] -> w_R/1
  [u_Sab] -> Calculo de Potencia eléctrica/1(u_Sab)
  [psi_Rab] -> Demux6/1
  [u_Sab] -> u_Sab/1
  Demux6/1 -> psi_Rab/1
  Calculo de Potencia eléctrica/3(i_S3abc) -> [i_S3abc]
  Demux6/2 -> psi_Rab/2
  Demux5/2 -> i_Sab/2
  [i_Sab] -> Calculo de Potencia eléctrica/2(i_Sab)
  [i_Sab] -> Demux5/1
  Demux/2 -> i_S3abc/2
  Demux3/1 -> u_S3abc/1
  Demux3/3 -> u_S3abc/3
  [i_S3abc] -> Demux/1
  Demux/1 -> i_S3abc/1
  Demux/3 -> i_S3abc/3
  [u_S3abc] -> Demux3/1
  Demux3/2 -> u_S3abc/2
  Modelo MI (Subsistema eléctrico)/1(i_Sab) -> [i_Sab]
  Modelo MI (Subsistema eléctrico)/3(tau_R) -> [tau_R]
  Product1/1 -> [P_mech]
  [w_R] -> Product1/1
  [tau_R] -> Product1/2
  [tau_R] -> Bus Creator/1  "tau_R"
  Sum1/1 -> Potencia/3
  [P_elect] -> Potencia/1, Sum1/1
  [P_mech] -> Potencia/2, Sum1/2
  [tau_R] -> tau_R/1
  dq/1 -> [w_R]
  [tau_Rref] -> Controlador PBC/1(tau_Rref)
  [w_R] -> Modelo MI (Subsistema eléctrico)/3(w_R)
  Bus Creator/1 -> To Workspace/1
  Constant1/1 -> [MI_motor_params]
  [tau_R] -> Scope/1
  Constant2/1 -> [PBC_params]
  [w_R] -> Bus Creator/2  "w_R"
  [u_Sab] -> Bus Creator/3  "u_Sab"
  [i_Sab] -> Bus Creator/4  "i_Sab"
  [u_S3abc] -> Bus Creator/5  "u_S3abc"
  [i_S3abc] -> Bus Creator/6  "i_S3abc"
  [P_elect] -> Bus Creator/7  "P_elect"
  [P_mech] -> Bus Creator/8  "P_mech"
  tau_Rref/1 -> [tau_Rref]

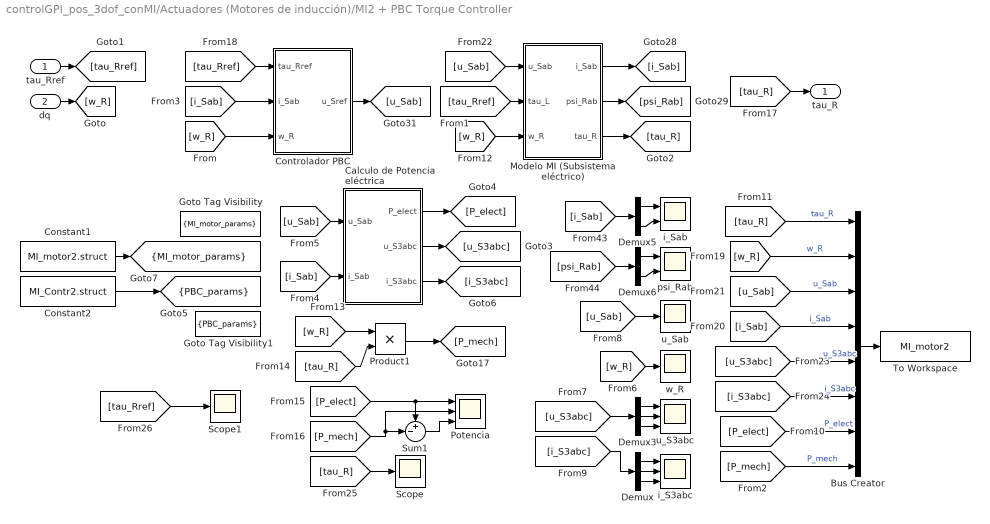
== system controlGPI_pos_3dof_conMI/Actuadores (Motores de inducción)/MI2 + PBC Torque Controller ==
  tau_Rref : Inport
  dq : Inport  Port=2
  Bus Creator : BusCreator  Inputs=8
  Calculo de Potencia eléctrica : Subsystem
  Constant1 : Constant  Value=MI_motor2.struct  OutDataTypeStr=Bus: MI_bus
  Constant2 : Constant  Value=MI_Contr2.struct  OutDataTypeStr=Bus: PBC_bus
  Controlador PBC : Subsystem
  Demux : Demux  Outputs=3
  Demux3 : Demux  Outputs=3
  Demux5 : Demux  Outputs=2
  Demux6 : Demux  Outputs=2
  Goto Tag Visibility : GotoTagVisibility  GotoTag=MI_motor_params
  Goto Tag Visibility1 : GotoTagVisibility  GotoTag=PBC_params
  Modelo MI (Subsistema eléctrico) : Subsystem
  Potencia : Scope  NumInputPorts=3
  Product1 : Product
  Scope : Scope
  Scope1 : Scope
  Sum1 : Sum  Inputs=+-|
  To Workspace : ToWorkspace  VariableName=MI_motor2  SaveFormat=Timeseries  SampleTime=-1
  i_S3abc : Scope  NumInputPorts=3
  i_Sab : Scope  NumInputPorts=2
  psi_Rab : Scope  NumInputPorts=2
  u_S3abc : Scope  NumInputPorts=3
  u_Sab : Scope
  w_R : Scope
  tau_R : Outport
  tag scope: MI_motor_params=scoped, PBC_params=scoped
  wires:
  Modelo MI (Subsistema eléctrico)/2(psi_Rab) -> [psi_Rab]
  [u_Sab] -> Modelo MI (Subsistema eléctrico)/1(u_Sab)
  [i_Sab] -> Controlador PBC/2(i_Sab)
  Controlador PBC/1(u_Sref) -> [u_Sab]
  [w_R] -> Controlador PBC/3(w_R)
  [tau_Rref] -> Modelo MI (Subsistema eléctrico)/2(tau_L)
  Calculo de Potencia eléctrica/2(u_S3abc) -> [u_S3abc]
  Calculo de Potencia eléctrica/1(P_elect) -> [P_elect]
  Demux5/1 -> i_Sab/1
  [w_R] -> w_R/1
  [u_Sab] -> Calculo de Potencia eléctrica/1(u_Sab)
  [psi_Rab] -> Demux6/1
  [u_Sab] -> u_Sab/1
  Demux6/1 -> psi_Rab/1
  Calculo de Potencia eléctrica/3(i_S3abc) -> [i_S3abc]
  Demux6/2 -> psi_Rab/2
  Demux5/2 -> i_Sab/2
  [i_Sab] -> Calculo de Potencia eléctrica/2(i_Sab)
  [i_Sab] -> Demux5/1
  Demux/2 -> i_S3abc/2
  Demux3/1 -> u_S3abc/1
  Demux3/3 -> u_S3abc/3
  [i_S3abc] -> Demux/1
  Demux/1 -> i_S3abc/1
  Demux/3 -> i_S3abc/3
  [u_S3abc] -> Demux3/1
  Demux3/2 -> u_S3abc/2
  Modelo MI (Subsistema eléctrico)/1(i_Sab) -> [i_Sab]
  Modelo MI (Subsistema eléctrico)/3(tau_R) -> [tau_R]
  Product1/1 -> [P_mech]
  [w_R] -> Product1/1
  [tau_R] -> Product1/2
  [tau_R] -> Bus Creator/1  "tau_R"
  Sum1/1 -> Potencia/3
  [P_elect] -> Potencia/1, Sum1/1
  [P_mech] -> Potencia/2, Sum1/2
  [tau_R] -> tau_R/1
  dq/1 -> [w_R]
  [tau_Rref] -> Controlador PBC/1(tau_Rref)
  [w_R] -> Modelo MI (Subsistema eléctrico)/3(w_R)
  Bus Creator/1 -> To Workspace/1
  Constant1/1 -> [MI_motor_params]
  [tau_R] -> Scope/1
  Constant2/1 -> [PBC_params]
  [w_R] -> Bus Creator/2  "w_R"
  [u_Sab] -> Bus Creator/3  "u_Sab"
  [i_Sab] -> Bus Creator/4  "i_Sab"
  [u_S3abc] -> Bus Creator/5  "u_S3abc"
  [i_S3abc] -> Bus Creator/6  "i_S3abc"
  [P_elect] -> Bus Creator/7  "P_elect"
  [P_mech] -> Bus Creator/8  "P_mech"
  [tau_Rref] -> Scope1/1
  tau_Rref/1 -> [tau_Rref]

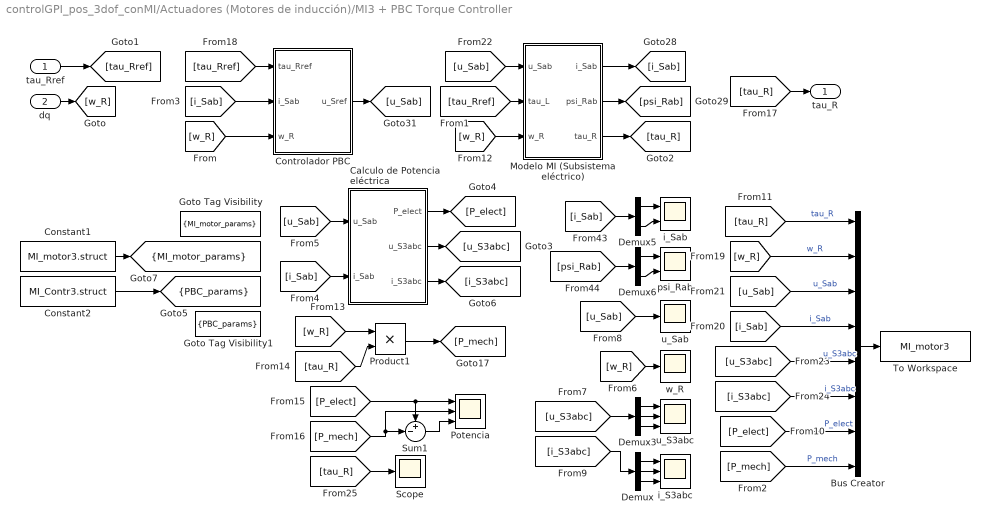
== system controlGPI_pos_3dof_conMI/Actuadores (Motores de inducción)/MI3 + PBC Torque Controller ==
  tau_Rref : Inport
  dq : Inport  Port=2
  Bus Creator : BusCreator  Inputs=8
  Calculo de Potencia eléctrica : Subsystem
  Constant1 : Constant  Value=MI_motor3.struct  OutDataTypeStr=Bus: MI_bus
  Constant2 : Constant  Value=MI_Contr3.struct  OutDataTypeStr=Bus: PBC_bus
  Controlador PBC : Subsystem
  Demux : Demux  Outputs=3
  Demux3 : Demux  Outputs=3
  Demux5 : Demux  Outputs=2
  Demux6 : Demux  Outputs=2
  Goto Tag Visibility : GotoTagVisibility  GotoTag=MI_motor_params
  Goto Tag Visibility1 : GotoTagVisibility  GotoTag=PBC_params
  Modelo MI (Subsistema eléctrico) : Subsystem
  Potencia : Scope  NumInputPorts=3
  Product1 : Product
  Scope : Scope
  Sum1 : Sum  Inputs=+-|
  To Workspace : ToWorkspace  VariableName=MI_motor3  SaveFormat=Timeseries  SampleTime=-1
  i_S3abc : Scope  NumInputPorts=3
  i_Sab : Scope  NumInputPorts=2
  psi_Rab : Scope  NumInputPorts=2
  u_S3abc : Scope  NumInputPorts=3
  u_Sab : Scope
  w_R : Scope
  tau_R : Outport
  tag scope: MI_motor_params=scoped, PBC_params=scoped
  wires:
  Modelo MI (Subsistema eléctrico)/2(psi_Rab) -> [psi_Rab]
  [u_Sab] -> Modelo MI (Subsistema eléctrico)/1(u_Sab)
  [i_Sab] -> Controlador PBC/2(i_Sab)
  Controlador PBC/1(u_Sref) -> [u_Sab]
  [w_R] -> Controlador PBC/3(w_R)
  [tau_Rref] -> Modelo MI (Subsistema eléctrico)/2(tau_L)
  Calculo de Potencia eléctrica/2(u_S3abc) -> [u_S3abc]
  Calculo de Potencia eléctrica/1(P_elect) -> [P_elect]
  Demux5/1 -> i_Sab/1
  [w_R] -> w_R/1
  [u_Sab] -> Calculo de Potencia eléctrica/1(u_Sab)
  [psi_Rab] -> Demux6/1
  [u_Sab] -> u_Sab/1
  Demux6/1 -> psi_Rab/1
  Calculo de Potencia eléctrica/3(i_S3abc) -> [i_S3abc]
  Demux6/2 -> psi_Rab/2
  Demux5/2 -> i_Sab/2
  [i_Sab] -> Calculo de Potencia eléctrica/2(i_Sab)
  [i_Sab] -> Demux5/1
  Demux/2 -> i_S3abc/2
  Demux3/1 -> u_S3abc/1
  Demux3/3 -> u_S3abc/3
  [i_S3abc] -> Demux/1
  Demux/1 -> i_S3abc/1
  Demux/3 -> i_S3abc/3
  [u_S3abc] -> Demux3/1
  Demux3/2 -> u_S3abc/2
  Modelo MI (Subsistema eléctrico)/1(i_Sab) -> [i_Sab]
  Modelo MI (Subsistema eléctrico)/3(tau_R) -> [tau_R]
  Product1/1 -> [P_mech]
  [w_R] -> Product1/1
  [tau_R] -> Product1/2
  [tau_R] -> Bus Creator/1  "tau_R"
  Sum1/1 -> Potencia/3
  [P_elect] -> Potencia/1, Sum1/1
  [P_mech] -> Potencia/2, Sum1/2
  [tau_R] -> tau_R/1
  dq/1 -> [w_R]
  [tau_Rref] -> Controlador PBC/1(tau_Rref)
  [w_R] -> Modelo MI (Subsistema eléctrico)/3(w_R)
  Bus Creator/1 -> To Workspace/1
  Constant1/1 -> [MI_motor_params]
  [tau_R] -> Scope/1
  Constant2/1 -> [PBC_params]
  [w_R] -> Bus Creator/2  "w_R"
  [u_Sab] -> Bus Creator/3  "u_Sab"
  [i_Sab] -> Bus Creator/4  "i_Sab"
  [u_S3abc] -> Bus Creator/5  "u_S3abc"
  [i_S3abc] -> Bus Creator/6  "i_S3abc"
  [P_elect] -> Bus Creator/7  "P_elect"
  [P_mech] -> Bus Creator/8  "P_mech"
  tau_Rref/1 -> [tau_Rref]

== system controlGPI_pos_3dof_conMI/ControladorGPI + NN/2 to 3 (1) ==
  In1 : Inport
  In2 : Inport  Port=2
  Demux : Demux  Outputs=3
  Demux1 : Demux  Outputs=3
  Mux : Mux  Inputs=2
  Mux1 : Mux  Inputs=2
  Mux2 : Mux  Inputs=2
  Out1 : Outport
  Out2 : Outport  Port=2
  Out3 : Outport  Port=3
  wires:
  Demux/3 -> Mux2/1
  Mux2/1 -> Out3/1
  Mux1/1 -> Out2/1
  Demux/1 -> Mux/1
  Demux1/1 -> Mux/2
  In1/1 -> Demux/1
  Demux/2 -> Mux1/1
  Demux1/2 -> Mux1/2
  Mux/1 -> Out1/1
  Demux1/3 -> Mux2/2
  In2/1 -> Demux1/1

== system controlGPI_pos_3dof_conMI/ControladorGPI + NN/3 to 9 (1) ==
  In1 : Inport
  In2 : Inport  Port=2
  In3 : Inport  Port=3
  Demux2 : Demux  Outputs=3
  Demux3 : Demux  Outputs=3
  Demux4 : Demux  Outputs=3
  Out1 : Outport
  Out2 : Outport  Port=2
  Out3 : Outport  Port=3
  Out4 : Outport  Port=4
  Out5 : Outport  Port=5
  Out6 : Outport  Port=6
  Out7 : Outport  Port=7
  Out8 : Outport  Port=8
  Out9 : Outport  Port=9
  wires:
  In3/1 -> Demux4/1
  Demux4/1 -> Out3/1
  Demux2/1 -> Out1/1
  Demux3/3 -> Out8/1
  Demux3/2 -> Out5/1
  Demux3/1 -> Out2/1
  In1/1 -> Demux2/1
  Demux2/3 -> Out7/1
  Demux4/3 -> Out9/1
  Demux4/2 -> Out6/1
  Demux2/2 -> Out4/1
  In2/1 -> Demux3/1

== system controlGPI_pos_3dof_conMI/ControladorGPI + NN/Red neuronal ==
  q : Inport
  de_q : Inport  Port=2
  e_p : Inport  Port=3
  B-Spline NNs : Subsystem  TreatAsAtomicUnit=on
  Constant3 : Constant  Value=nn_select
  Constants : Subsystem  TreatAsAtomicUnit=on
  GPI_params : Scope  NumInputPorts=3
  Merge : Merge  Inputs=3
  Merge1 : Merge  Inputs=3
  Merge2 : Merge  Inputs=3
  RBF NNs : Subsystem  TreatAsAtomicUnit=on
  nn_select : Display
  param sintonization selector : If  IfExpression=u1 == 1  ElseIfExpressions=u1 == 2
  Wc : Outport
  Zc : Outport  Port=2
  Pc : Outport  Port=3
  wires:
  param sintonization selector/1 -> B-Spline NNs/Action
  B-Spline NNs/1(Wc) -> Merge/1
  param sintonization selector/3 -> Constants/Action
  Constant3/1 -> nn_select/1, param sintonization selector/1
  B-Spline NNs/2(Zc) -> Merge1/1
  B-Spline NNs/3(Pc) -> Merge2/1
  Constants/1(Wc) -> Merge/2
  Constants/2(Zc) -> Merge1/2
  Constants/3(Pc) -> Merge2/2
  q/1 -> [e_q]
  de_q/1 -> [de_q]
  param sintonization selector/2 -> RBF NNs/Action
  RBF NNs/2(Zc) -> Merge1/3
  RBF NNs/1(Wc) -> Merge/3
  RBF NNs/3(Pc) -> Merge2/3
  Merge/1 -> GPI_params/1, Wc/1
  Merge1/1 -> GPI_params/2, Zc/1
  Merge2/1 -> GPI_params/3, Pc/1
  [e_q] -> B-Spline NNs/1(e_q)
  [de_q] -> B-Spline NNs/2(de_q)
  [e_q] -> RBF NNs/1(e_q)
  [de_q] -> RBF NNs/2(de_q)
  e_p/1 -> [e_p]
  [e_p] -> RBF NNs/3(e_p)
  [e_p] -> B-Spline NNs/3(e_p)

== system controlGPI_pos_3dof_conMI/Perfil torque de carga tau_L/If Action Subsystem ==
  perfil_params : Inport
  Action Port : ActionPort
  Clock2 : Clock
  Clock4 : Clock
  Polinomio 7mo orden sen : MATLAB Function  TreatAsAtomicUnit=on
  Scope1 : Scope
  Scope4 : Scope
  Scope5 : Scope  NumInputPorts=4
  Senoidal tiempo de inicio : MATLAB Function  TreatAsAtomicUnit=on
  Sum1 : Sum  Inputs=|-+
  senoidal : Sin  TimeSource=Use external signal  Frequency=6.2832  Phase=1.5708  SampleTime=0
  sen : Outport
  wires:
  Clock4/1 -> Polinomio 7mo orden sen/1(t)
  Polinomio 7mo orden sen/1(qpol) -> Scope1/1, Sum1/1, Scope5/1
  Sum1/1 -> Scope4/1, [sen]
  Polinomio 7mo orden sen/4(jpol) -> Scope5/4
  Polinomio 7mo orden sen/3(apol) -> Scope5/3
  Clock2/1 -> Senoidal tiempo de inicio/1(t)
  [perfil_params] -> Polinomio 7mo orden sen/2(perfil_params)
  Polinomio 7mo orden sen/2(vpol) -> Scope5/2
  senoidal/1 -> Sum1/2
  Senoidal tiempo de inicio/1(tr) -> senoidal/1
  [sen] -> sen/1
  perfil_params/1 -> [perfil_params]
  [perfil_params] -> Senoidal tiempo de inicio/2(perfil_params)

== system controlGPI_pos_3dof_conMI/Perfil torque de carga tau_L/If Action Subsystem1 ==
  Action Port : ActionPort
  Constant : Constant  Value=0
  cero : Outport
  wires:
  Constant/1 -> cero/1

== system controlGPI_pos_3dof_conMI/Perfil torque de carga tau_L/If Action Subsystem2 ==
  Action Port : ActionPort
  Scope3 : Scope
  Sum : Sum  Inputs=|++
  escalon1 : Step  Time=2.5  After=0.70582  SampleTime=0
  escalon2 : Step  Time=7.5  After=-0.70582  SampleTime=0
  esca : Outport
  wires:
  escalon2/1 -> Sum/2
  escalon1/1 -> Sum/1
  Sum/1 -> [esca], Scope3/1
  [esca] -> esca/1

== system controlGPI_pos_3dof_conMI/Perfil torque de carga tau_L/If Action Subsystem3 ==
  Action Port : ActionPort
  Scope2 : Scope
  Sum2 : Sum  Inputs=|++
  rampa1 : simulink/Sources/Ramp  slope=0.02064  start=2.5  InitialOutput=0
  rampa2 : simulink/Sources/Ramp  slope=-0.02064  start=7.5  InitialOutput=0
  ramp : Outport
  wires:
  rampa2/1 -> Sum2/2
  rampa1/1 -> Sum2/1
  Sum2/1 -> Scope2/1, [ramp]
  [ramp] -> ramp/1

== system controlGPI_pos_3dof_conMI/Perfil torque de carga tau_L/If Action Subsystem4 ==
  perfil_params : Inport
  Action Port : ActionPort
  Clock1 : Clock
  Polinomio 7mo orden tau_L : MATLAB Function  TreatAsAtomicUnit=on
  Scope : Scope  NumInputPorts=4
  pol7 : Outport
  wires:
  Polinomio 7mo orden tau_L/4(jpol) -> Scope/4
  Polinomio 7mo orden tau_L/1(qpol) -> Scope/1, [pol7]
  Polinomio 7mo orden tau_L/2(vpol) -> Scope/2
  Clock1/1 -> Polinomio 7mo orden tau_L/1(t)
  Polinomio 7mo orden tau_L/3(apol) -> Scope/3
  perfil_params/1 -> Polinomio 7mo orden tau_L/2(perfil_params)
  [pol7] -> pol7/1

== system controlGPI_pos_3dof_conMI/Perfil torque de carga tau_L/If Action Subsystem5 ==
  perfil_params : Inport
  Action Port : ActionPort
  Clock : Clock
  Scope1 : Scope
  Tren de esca : MATLAB Function  TreatAsAtomicUnit=on
  trEsca : Outport
  wires:
  Tren de esca/1(q) -> Scope1/1, [trEsca]
  Clock/1 -> Tren de esca/1(t)
  perfil_params/1 -> Tren de esca/2(perfil_params)
  [trEsca] -> trEsca/1

== system controlGPI_pos_3dof_conMI/Perfil torque de carga tau_L/If Action Subsystem6 ==
  Action Port : ActionPort
  Clock3 : Clock
  Polinomio 7mo orden timeseries : MATLAB Function  TreatAsAtomicUnit=on
  Product : Product
  Scope6 : Scope  NumInputPorts=4
  ts_data1 : FromWorkspace  Commented=on  VariableName=tau_L_ts
  ts : Outport
  wires:
  Product/1 -> [ts]
  Clock3/1 -> Polinomio 7mo orden timeseries/1(t)
  ts_data1/1 -> Product/1
  Polinomio 7mo orden timeseries/4(jpol) -> Scope6/4
  Polinomio 7mo orden timeseries/2(vpol) -> Scope6/2
  Polinomio 7mo orden timeseries/3(apol) -> Scope6/3
  Polinomio 7mo orden timeseries/1(qpol) -> Product/2, Scope6/1
  [ts] -> ts/1

== system controlGPI_pos_3dof_conMI/Perfil torque de carga tau_L/If Action Subsystem7 ==
  perfil_params : Inport
  Action Port : ActionPort
  Clock5 : Clock
  Scope7 : Scope
  Trayectoria 15 segmentos : MATLAB Function  TreatAsAtomicUnit=on
  tr15segs : Outport
  wires:
  Clock5/1 -> Trayectoria 15 segmentos/1(t)
  Trayectoria 15 segmentos/1(q) -> Scope7/1, [tr15segs]
  [tr15segs] -> tr15segs/1
  perfil_params/1 -> Trayectoria 15 segmentos/2(perfil_params)

== system controlGPI_pos_3dof_conMI/Trayectoria de referencia/2 to 3 (2) ==
  In1 : Inport
  In2 : Inport  Port=2
  Demux3 : Demux  Outputs=3
  Demux4 : Demux  Outputs=3
  Mux10 : Mux  Inputs=2
  Mux8 : Mux  Inputs=2
  Mux9 : Mux  Inputs=2
  1 : Outport
  2 : Outport  Port=2
  3 : Outport  Port=3
  wires:
  Demux4/3 -> Mux10/2
  Demux3/1 -> Mux8/1
  Demux3/2 -> Mux9/1
  Mux9/1 -> 2/1
  Demux4/2 -> Mux9/2
  Demux4/1 -> Mux8/2
  Demux3/3 -> Mux10/1
  Mux8/1 -> 1/1
  Mux10/1 -> 3/1
  In1/1 -> Demux3/1
  In2/1 -> Demux4/1

== system controlGPI_pos_3dof_conMI/Trayectoria de referencia/2 to 3 (2)1 ==
  In1 : Inport
  In2 : Inport  Port=2
  Demux3 : Demux  Outputs=3
  Demux4 : Demux  Outputs=3
  Mux10 : Mux  Inputs=2
  Mux8 : Mux  Inputs=2
  Mux9 : Mux  Inputs=2
  1 : Outport
  2 : Outport  Port=2
  3 : Outport  Port=3
  wires:
  Demux4/3 -> Mux10/2
  Demux3/1 -> Mux8/1
  Demux3/2 -> Mux9/1
  Mux9/1 -> 2/1
  Demux4/2 -> Mux9/2
  Demux4/1 -> Mux8/2
  Demux3/3 -> Mux10/1
  Mux8/1 -> 1/1
  Mux10/1 -> 3/1
  In1/1 -> Demux3/1
  In2/1 -> Demux4/1

== system controlGPI_pos_3dof_conMI/Trayectoria de referencia/2 to 3 (2)2 ==
  In1 : Inport
  In2 : Inport  Port=2
  Demux3 : Demux  Outputs=3
  Demux4 : Demux  Outputs=3
  Mux10 : Mux  Inputs=2
  Mux8 : Mux  Inputs=2
  Mux9 : Mux  Inputs=2
  1 : Outport
  2 : Outport  Port=2
  3 : Outport  Port=3
  wires:
  Demux4/3 -> Mux10/2
  Demux3/1 -> Mux8/1
  Demux3/2 -> Mux9/1
  Mux9/1 -> 2/1
  Demux4/2 -> Mux9/2
  Demux4/1 -> Mux8/2
  Demux3/3 -> Mux10/1
  Mux8/1 -> 1/1
  Mux10/1 -> 3/1
  In1/1 -> Demux3/1
  In2/1 -> Demux4/1

== system controlGPI_pos_3dof_conMI/Trayectoria de referencia/3 to 9 (1)1 ==
  In1 : Inport
  In2 : Inport  Port=2
  In3 : Inport  Port=3
  Demux2 : Demux  Outputs=3
  Demux3 : Demux  Outputs=3
  Demux4 : Demux  Outputs=3
  Out1 : Outport
  Out2 : Outport  Port=2
  Out3 : Outport  Port=3
  Out4 : Outport  Port=4
  Out5 : Outport  Port=5
  Out6 : Outport  Port=6
  Out7 : Outport  Port=7
  Out8 : Outport  Port=8
  Out9 : Outport  Port=9
  wires:
  In3/1 -> Demux4/1
  Demux4/1 -> Out3/1
  Demux2/1 -> Out1/1
  Demux3/3 -> Out8/1
  Demux3/2 -> Out5/1
  Demux3/1 -> Out2/1
  In1/1 -> Demux2/1
  Demux2/3 -> Out7/1
  Demux4/3 -> Out9/1
  Demux4/2 -> Out6/1
  Demux2/2 -> Out4/1
  In2/1 -> Demux3/1

== system controlGPI_pos_3dof_conMI/Trayectoria de referencia/3 to 9 (7) ==
  In1 : Inport
  In2 : Inport  Port=2
  In3 : Inport  Port=3
  Demux2 : Demux  Outputs=3
  Demux3 : Demux  Outputs=3
  Demux4 : Demux  Outputs=3
  Out1 : Outport
  Out2 : Outport  Port=2
  Out3 : Outport  Port=3
  Out4 : Outport  Port=4
  Out5 : Outport  Port=5
  Out6 : Outport  Port=6
  Out7 : Outport  Port=7
  Out8 : Outport  Port=8
  Out9 : Outport  Port=9
  wires:
  In3/1 -> Demux4/1
  Demux4/1 -> Out3/1
  Demux2/1 -> Out1/1
  Demux3/3 -> Out8/1
  Demux3/2 -> Out5/1
  Demux3/1 -> Out2/1
  In1/1 -> Demux2/1
  Demux2/3 -> Out7/1
  Demux4/3 -> Out9/1
  Demux4/2 -> Out6/1
  Demux2/2 -> Out4/1
  In2/1 -> Demux3/1

== system controlGPI_pos_3dof_conMI/Trayectoria de referencia/Inicializar posición de robot manipulador ==
  q_r : Inport
  2 to 3 (3) : Subsystem
  Clock1 : Clock
  Constant : Constant  Value=q0
  Constant1 : Constant  Value=q_eq
  Constant2 : Constant  Value=tr_muestra
  Constant3 : Constant  Value=ndof
  Constant4 : Constant  Value=t_qeq_init
  Constant5 : Constant  Value=t_trtr
  Constant7 : Constant  Value=t_tr_init
  Demux{1..4} (4 alike) : Demux  Outputs=3
  Derivative : Derivative
  Derivative1 : Derivative
  ddq_ref1 : Scope  NumInputPorts=3
  dq_ref1 : Scope  NumInputPorts=3
  interp_pol7_q_r : MATLAB Function  TreatAsAtomicUnit=on
  q_r1 : Scope  NumInputPorts=3
  q_r_comp : Scope  NumInputPorts=3
  q_ref1 : Scope  NumInputPorts=3
  q_ref : Outport
  dq_ref : Outport  Port=2
  ddq_ref : Outport  Port=3
  wires:
  [ddq_ref] -> ddq_ref/1
  q_r/1 -> [q_r]
  [dq_ref] -> dq_ref/1
  [q_ref] -> q_ref/1
  [q_r] -> 2 to 3 (3)/1(In1)
  [q_ref] -> 2 to 3 (3)/2(In2)
  [q_r] -> Demux3/1
  interp_pol7_q_r/1(interp_qpos) -> [q_ref], Derivative/1
  Derivative/1 -> [dq_ref], Derivative1/1
  Derivative1/1 -> [ddq_ref]
  [q_ref] -> Demux1/1
  [dq_ref] -> Demux2/1
  [ddq_ref] -> Demux4/1
  Demux3/2 -> q_r1/2
  Demux3/1 -> q_r1/1
  Demux3/3 -> q_r1/3
  Demux1/2 -> q_ref1/2
  Demux1/1 -> q_ref1/1
  Demux1/3 -> q_ref1/3
  Demux2/2 -> dq_ref1/2
  Demux2/1 -> dq_ref1/1
  Demux2/3 -> dq_ref1/3
  Demux4/2 -> ddq_ref1/2
  Demux4/1 -> ddq_ref1/1
  Demux4/3 -> ddq_ref1/3
  2 to 3 (3)/3(3) -> q_r_comp/3
  2 to 3 (3)/1(1) -> q_r_comp/1
  2 to 3 (3)/2(2) -> q_r_comp/2
  Constant5/1 -> interp_pol7_q_r/7(t_trtr)
  Constant4/1 -> interp_pol7_q_r/5(t0)
  Constant1/1 -> interp_pol7_q_r/2(q_eq)
  [q_r] -> interp_pol7_q_r/4(q_tr_init)
  Constant3/1 -> interp_pol7_q_r/9(ndof)
  Constant/1 -> interp_pol7_q_r/3(q_cero)
  Clock1/1 -> interp_pol7_q_r/1(t)
  Constant7/1 -> interp_pol7_q_r/6(t1)
  Constant2/1 -> interp_pol7_q_r/8(tr_muestra)
